simulink model "非线性系统simulink仿真"  (R2016b)
settings: Solver=VariableStepAuto  StartTime=0.0  StopTime=10  FixedStep=0.1  RelTol=1e-3
libraries: simulink x1
settings Model: Creator=Jake  LastModifiedBy=Jake

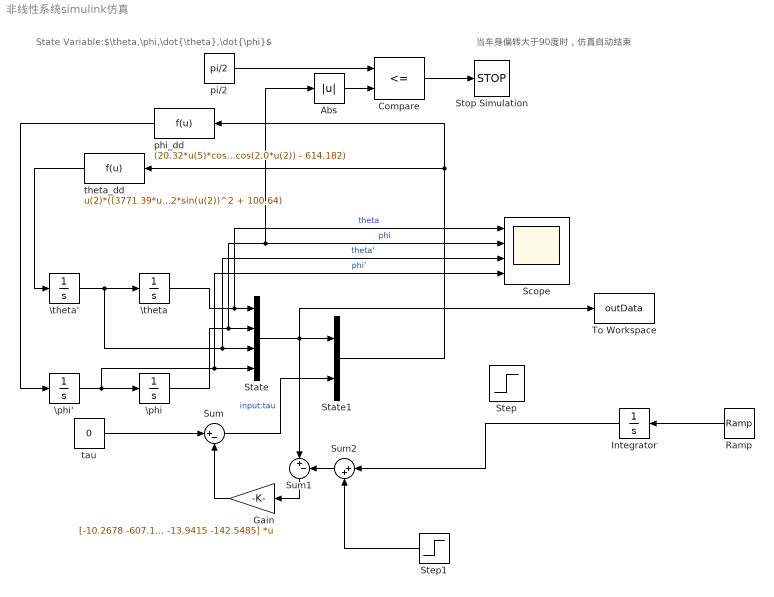
== system 非线性系统simulink仿真 ==
  note: State Variable:$\theta,\phi,\dot{\theta},\dot{\phi}$
  note: 当车身偏转大于90度时，仿真自动结束
  Abs : Abs
  Compare : RelationalOperator  Operator=<=  OutDataTypeStr=boolean  RndMeth=Simplest
  Gain : Gain  Gain="[-10.2678 -607.1284  -13.9415 -142.5485]"  Multiplication=Matrix(K*u)
  Integrator : Integrator
  Ramp : simulink/Sources/Ramp  slope=[1 0 0 0]  start=0  X0=0
  Scope : Scope  NumInputPorts=4
  State : Concatenate  NumInputs=4
  State1 : Concatenate
  Step : Step  Time=2  After=[0 0.1 0 0]  SampleTime=0
  Step1 : Step  Time=6  After=[0 0 0 0]  SampleTime=0
  Stop Simulation : Stop
  Sum : Sum  Inputs=|+-
  Sum1 : Sum  Inputs=|+-
  Sum2 : Sum  Inputs=|++
  To Workspace : ToWorkspace  VariableName=outData  SaveFormat=Structure With Time  SampleTime=-1
  \phi : Integrator
  \phi' : Integrator
  \theta : Integrator
  \theta' : Integrator
  phi_dd : Fcn  Expr=(20.32*u(5)*cos(u(2)))/(412.902*cos(u(2))^2 - 513.542) - 1.0*u(2)*((825.805*cos(2.0*u(2))*u(4)^2 + 8678.42*cos(u(2)) + 40.64*u(5)*sin(u(2)) - 3.2512*u(3)*sin(u(2)))/(412.902*cos(2.0*u(2)) - 614.182) + (132129.0*sin(2.0*u(2))*(2.58064*sin(2.0*u(2))*u(4)^2 + 54.2401*sin(u(2)) - 0.254*u(5)*cos(u(2)) + 0.02032*u(3)*cos(u(2))))/(412.902*cos(2.0*u(2)) - 614.182)^2) - (1.6256*u(3)*cos(u(2)))/(412.902*cos(u(2))^2 - 513.542) - (825.805*u(4)^2*sin(2.0*u(2)))/(412.902*cos(2.0*u(2)) - 614.182)
  pi/2 : Constant  Value=pi/2
  tau : Constant  Value=0
  theta_dd : Fcn  Expr=u(2)*((3771.39*u(4)^2*cos(u(2)) + 63733.3*cos(u(2))^2 - 31866.6)/(825.805*cos(u(2))^2 - 1027.08) + (1651.61*sin(2.0*u(2))*(1885.7*sin(u(2))*u(4)^2 - 92.8*u(5) + 7.424*u(3) + 7966.66*sin(2.0*u(2))))/(412.902*cos(2.0*u(2)) - 614.182)^2) - (92.8*u(5))/(412.902*cos(u(2))^2 - 513.542) + (7.424*u(3))/(412.902*cos(u(2))^2 - 513.542) - (3771.39*u(4)^2*sin(u(2)))/(412.902*sin(u(2))^2 + 100.64)
  wires:
  \theta'/1 -> Scope/3, State/3, \theta/1  "theta'"
  \phi'/1 -> Scope/4, State/4, \phi/1  "phi'"
  \theta/1 -> Scope/1, State/1  "theta"
  \phi/1 -> Abs/1, Scope/2, State/2  "phi"
  theta_dd/1 -> \theta'/1
  phi_dd/1 -> \phi'/1
  Gain/1 -> Sum/2
  Sum/1 -> State1/2  "input:tau"
  tau/1 -> Sum/1
  Sum1/1 -> Gain/1
  Sum2/1 -> Sum1/2
  Step1/1 -> Sum2/2
  State1/1 -> theta_dd/1, phi_dd/1
  Compare/1 -> Stop Simulation/1
  pi/2/1 -> Compare/1
  Abs/1 -> Compare/2
  State/1 -> Sum1/1, To Workspace/1, State1/1
  Ramp/1 -> Integrator/1
  Integrator/1 -> Sum2/1
